simulink model "Project_sim"  (R2025b)
settings: Solver=ode4  StartTime=0.0  StopTime=2*T  FixedStep=0.1  RelTol=1e-3
values from neighbouring files (symbols this model uses):
  a = 3000+R_E    [RUN_ME.m]
  A_0 = [cos(th0+epsilon1) sin(th0+epsilon1) 0; -sin(th0+epsilon1) cos(th0+epsilon1) 0; 0 0 1]*    [1 0 0; 0 cos(i+epsilon2) sin(i+epsilon2); 0 -sin(i+epsilon2) cos(i+epsilon2)]    [RUN_ME.m]
  alpha1 = 0.72    [RUN_ME.m]
  alpha_G0 = 0    [RUN_ME.m]
  AU = astroConstants(2)    [RUN_ME.m]
  b_gyro = deg2rad(0.01*rand(1))    [RUN_ME.m]
  b_mag = 15e-9    (= 1.5e-08)    [RUN_ME.m]
  b_sun = deg2rad(0.1*rand(1))    [RUN_ME.m]
  c_time = 100    [RUN_ME.m]
  D = zeros(3)    [RUN_ME.m]
  den_cz_mag = double(sym2poly(den8_z_mag))    [RUN_ME.m]
  den_cz_sun = double(sym2poly(den8_z_sun))    [RUN_ME.m]
  e = 0.2    [RUN_ME.m]
  epsilon = astroConstants(8)    [RUN_ME.m]
  g_IGRF = [ ... (first row only)    [RUN_ME.m]
  gyro_delay = 1    [RUN_ME.m]
  gyro_mounting = eye(3)    [RUN_ME.m]
  h_IGRF = [ ... (first row only)    [RUN_ME.m]
  I = [Ix 0 0; 0 Iy 0; 0 0 Iz]    [RUN_ME.m]
  i = deg2rad(30)    [RUN_ME.m]
  j_B = [0.01; 0.05; 0.01]    [RUN_ME.m]
  K = place(A, -B, a_controlled)    [RUN_ME.m]
  k1 = 20e-4    (= 0.002)    [RUN_ME.m]
  k1_tilde = 5e-4    (= 0.0005)    [RUN_ME.m]
  k2 = 2e-4    (= 0.0002)    [RUN_ME.m]
  Mis_gyro = deg2rad(0.1*rand(3,1))    [RUN_ME.m]
  Mis_mag = deg2rad(0.1*rand(3,1))    [RUN_ME.m]
  Mis_sun = deg2rad(0.1*rand(3,1))    [RUN_ME.m]
  mu = astroConstants(13)    [RUN_ME.m]
  n = sqrt(mu/a^3)    [RUN_ME.m]
  noise_density_mag = 16e-9    (= 1.6e-08)    [RUN_ME.m]
  Nonorthog_err_gyro = deg2rad(0.1*rand(3,1))    [RUN_ME.m]
  Nonorthog_err_mag = deg2rad(1)*ones(3,1)    [RUN_ME.m]
  num_cz_mag = double(sym2poly(num8_z_mag))    [RUN_ME.m]
  num_cz_sun = double(sym2poly(num8_z_sun))    [RUN_ME.m]
  R_E = astroConstants(23)    [RUN_ME.m]
  R_sun = astroConstants(3)    [RUN_ME.m]
  saturation_gyro = deg2rad(100)    [RUN_ME.m]
  saturation_mag = 60e-6    (= 6e-05)    [RUN_ME.m]
  SF = deg2rad(20*5.25e-3)    [RUN_ME.m]
  SFn = 0.02/100    (= 0.0002)    [RUN_ME.m]
  sigma_ARW = ARW/sqrt(Ts_gyro)    [RUN_ME.m]
  sigma_bias = bias_instability/sqrt(Ts_gyro)    [RUN_ME.m]
  sigma_RRW = RRW/sqrt(Ts_gyro)    [RUN_ME.m]
  sigma_sun = deg2rad(0.5)    [RUN_ME.m]
  th0 = deg2rad(0)    [RUN_ME.m]
  Ts = 0.1    [RUN_ME.m]
  Ts_gyro = 0.1    [RUN_ME.m]
  Ts_mag = 0.1    [RUN_ME.m]
  Ts_sun = 0.1    [RUN_ME.m]
  w_E = 2*pi/T_E    [RUN_ME.m]
  wx_0 = rand(1)*pi/6    [RUN_ME.m]
  wy_0 = rand(1)*pi/6    [RUN_ME.m]
  wz_0 = rand(1)*pi/6    [RUN_ME.m]
undefined symbols (not defined in the file or in its folder): DiscIntNeverNeededParam, dspblkCoreblockFVToolHelper, gcbh, magnitude, precision_sun, RW
libraries: Lib_rotation_matrix x17, matrix_library x11, simulink x3
(part 3 of 3)

== matlab function Project_sim/Environment/MATLAB Function1 ==
  data: r_N input; N input; R input; g_DGRF input; h_DGRF input; alpha_G_0 input; B_N output; w_E input; t input
function B_N = fcn(r_N, N, R, g_DGRF, h_DGRF, alpha_G_0, w_E, t)

z = r_N(3,1);
x = r_N(1,1);
y = r_N(2,1);
r = norm(r_N);

alpha = atan2(y/r, x/r);
delta = asin(z/r);
theta = pi/2 - delta;
alpha_G = alpha_G_0 + t * w_E;

% if (y/r) > 0
%     alpha = acos((x/r)/cos(delta));
% else
%     alpha = 2*pi - acos((x/r)/cos(delta));
% end

phi = alpha - alpha_G;

% Schmidt quasi-normalization factors

S = zeros (N+1, N+1); % S_i,j = S(i + 1, j + 1)
S(1,1) = 1;

% Associated Legendre Polynomials

P = zeros (N+1, N+1); % P_i,j = P(i + 1, j + 1)
P (1,1) = 1;

% Derivatives of associated Legendre polynomials

dP = zeros (N+1, N+1); % dP_i,j = dP(i + 1, j + 1)
dP(1,1) = 0;

% Compute Schmidt quasi-normalization factors

for n = 1:N
    for m = 0:n
        if (m == 0)
            S(n+1, 1) = S(n, 1)*(2*n-1)/n;
        else
            S(n+1, m+1) = S(n+1, m)*sqrt((n-m+1)*((m == 1) + 1)/(n + m));
        end
    end
end

% Compute associated Legendre Polynomials and derivatives of associated Legendre polynomials

for n = 1:N
    for m = 0:n
        if (n == 1)
            k = 0;
        else
            k = ((n - 1)^2 - m^2)/((2*n - 1)*(2*n -3));
        end

        if (n == m)
            P(n+1, m+1) = sin(theta)*P(n, m);
            dP(n+1, m+1) = sin(theta)*dP(n, m) + cos(theta)*P(n, m);
        elseif (n == 1)
            P(n+1, m+1) = cos(theta)*P(n, m+1);
            dP(n+1, m+1) = cos(theta)*dP(n, m+1) - sin(theta)*P(n, m+1);
        else
            P(n+1, m+1) = cos(theta)*P(n, m+1) - k*P(n-1, m+1);
            dP(n+1, m+1) = cos(theta)*dP(n, m+1) - sin(theta)*P(n, m+1) - k*dP(n-1, m+1);
        end
    end
end

% Compute quasi-normalized associated Legendre polynomials
% 
Pqn = S.*P;
dPqn = S.*dP;

% Gaussian coefficients are already Schmidt semi-normalized

% g_DGRFn = S(2:N+1, :).*g_DGRF(1:N, 1:N+1);
% h_DGRFn = S(2:N+1, :).*h_DGRF(1:N, 1:N+1);
g_DGRFn = g_DGRF;
h_DGRFn = h_DGRF;

% Initialize magnetic field components

b_r = 0;
b_theta = 0;
b_phi = 0;

% Compute magnetic field

for n = 1:N

    b_r_temp = 0;
    b_theta_temp = 0;
    b_phi_temp = 0;

    for m = 0:n
        b_r_temp = b_r_temp + (g_DGRFn(n, m+1)*cos(m*phi) + h_DGRFn(n, m+1)*sin(m*phi))*Pqn(n+1, m+1);
        b_theta_temp = b_theta_temp + (g_DGRFn(n, m+1)*cos(m*phi) + h_DGRFn(n, m+1)*sin(m*phi))*dPqn(n+1, m+1);
        b_phi_temp = b_phi_temp + m*(-g_DGRFn(n, m+1)*sin(m*phi) + h_DGRFn(n, m+1)*cos(m*phi))*Pqn(n+1, m+1);
    end

    b_r = b_r + b_r_temp*(n+1)*(R/r)^(n+2);
    b_theta = b_theta + b_theta_temp*(R/r)^(n+2);
    b_phi = b_phi + b_phi_temp*(R/r)^(n+2);

end

b_r = -b_r;
b_theta = -b_theta;
b_phi = -1/sin(theta)*b_phi;

b = [b_r; b_theta; b_phi];

R = [cos(delta)*cos(alpha), sin(delta)*cos(alpha), -sin(alpha);
    cos(delta)*sin(alpha), sin(delta)*sin(alpha), cos(alpha);
    sin(delta), cos(delta), 0];

B_N = R*b;

% B_1 = (b_r*cos(delta) + b_theta*sin(delta))*cos(alpha) - b_phi*sin(alpha);
% B_2 = (b_r*cos(delta) + b_theta*sin(delta))*sin(alpha) + b_phi*cos(alpha);
% B_3 = (b_r*sin(delta) - b_theta*cos(delta));
% B_N = [B_1; B_2; B_3];
